simulink model "WindowsiCreateNew"  (R2013a)
settings: Solver=ode3  StartTime=0.0  StopTime=inf  FixedStep=0.01  RelTol=1e-3
undefined symbols (not defined in the file): serial
libraries: instrumentlib x2, vrlib x1, aerolibanimutils x1
settings Model: Creator=Admin  LastModifiedBy=Admin

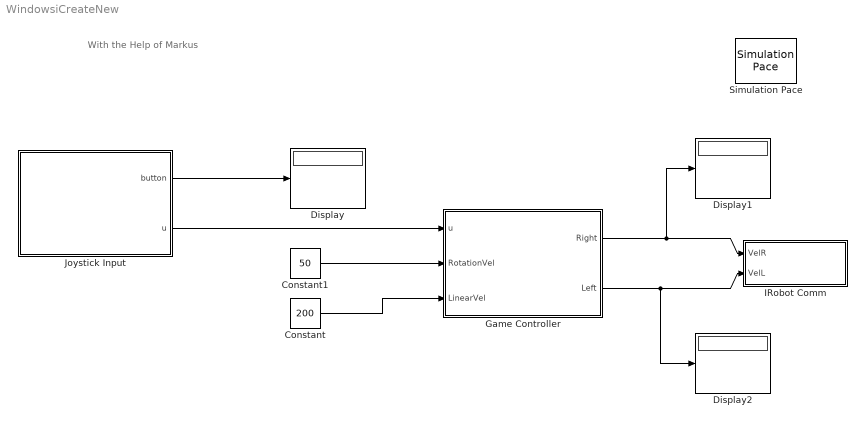
== system WindowsiCreateNew ==
  note: With the Help of Markus
  Constant : Constant  Value=200
  Constant1 : Constant  Value=50
  Display : Display
  Display1 : Display
  Display2 : Display
  Game Controller : MATLAB Function  TreatAsAtomicUnit=on
  IRobot Comm : Subsystem
  Joystick Input : Subsystem
  Simulation Pace : aerolibanimutils/Simulation Pace  SimulationPace=1  SleepMode=MATLAB Thread  OutputPaceError=off  SampleTime=-1
      settings: AttributesFormatString=%<SimulationPace> sec/sec
  wires:
  Joystick Input/1(button) -> Display/1
  Joystick Input/2(u) -> Game Controller/1(u)
  Game Controller/1(Right) -> Display1/1, IRobot Comm/1(VelR)
  Game Controller/2(Left) -> Display2/1, IRobot Comm/2(VelL)
  Constant1/1 -> Game Controller/2(RotationVel)
  Constant/1 -> Game Controller/3(LinearVel)

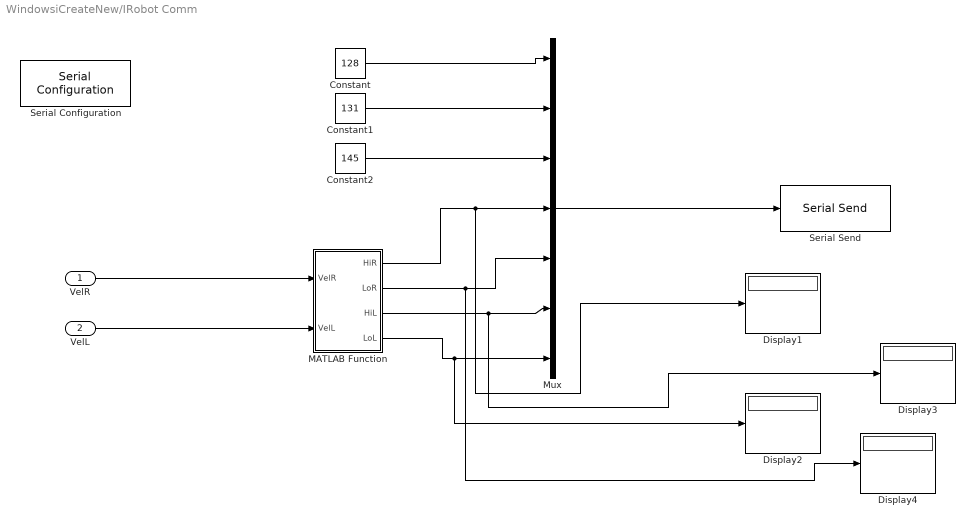
== system WindowsiCreateNew/IRobot Comm ==
  VelR : Inport
  VelL : Inport  Port=2
  Constant : Constant  Value=128  OutDataTypeStr=uint8
  Constant1 : Constant  Value=131  OutDataTypeStr=uint8
  Constant2 : Constant  Value=145  OutDataTypeStr=uint8
  Display{1..4} (4 alike) : Display
  MATLAB Function : MATLAB Function  TreatAsAtomicUnit=on
  Mux : Mux  Inputs=7
  Serial Configuration : instrumentlib/Serial Configuration  Priority=-200000  ComPortMenu=<Please select a port...>  ComPort=COM4  ObjConstructor=serial('COM4');  BaudRate=57600  DataBits=8  Parity=none  StopBits=1  FlowControl=none  Timeout=10  ByteOrder=LittleEndian
  Serial Send : instrumentlib/Serial Send  ComPortMenu=<Please select a port...>  ComPort=COM4  ObjConstructor=serial('COM4');  Terminator=<none>  EnableBlockingMode=off
  wires:
  MATLAB Function/1(HiR) -> Display1/1, Mux/4
  MATLAB Function/2(LoR) -> Display4/1, Mux/5
  MATLAB Function/3(HiL) -> Display3/1, Mux/6
  MATLAB Function/4(LoL) -> Display2/1, Mux/7
  Mux/1 -> Serial Send/1
  VelR/1 -> MATLAB Function/1(VelR)
  VelL/1 -> MATLAB Function/2(VelL)
  Constant/1 -> Mux/1
  Constant1/1 -> Mux/2
  Constant2/1 -> Mux/3

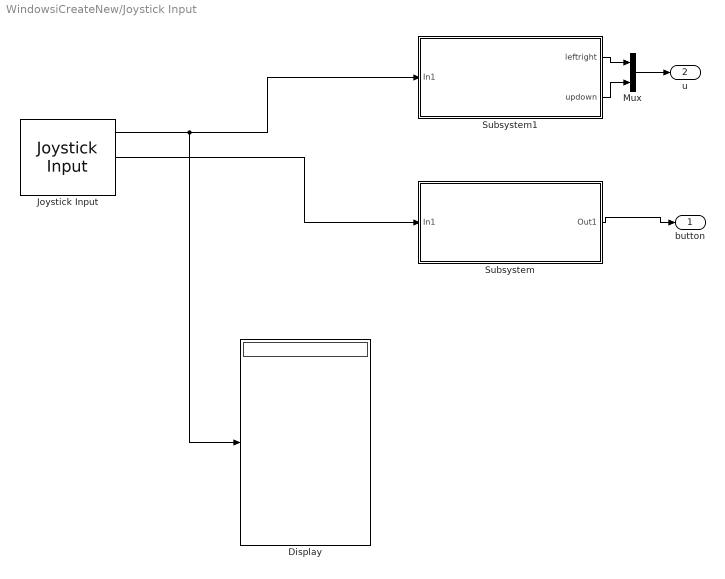
== system WindowsiCreateNew/Joystick Input ==
  Display : Display
  Joystick Input : vrlib/Joystick Input  joyid=1  adjustports=on  forcefeed=off
  Mux : Mux  Inputs=2
  Subsystem : Subsystem
  Subsystem1 : Subsystem
  button : Outport
  u : Outport  Port=2
  wires:
  Subsystem/1(Out1) -> button/1
  Mux/1 -> u/1
  Subsystem1/1(leftright) -> Mux/1
  Subsystem1/2(updown) -> Mux/2
  Joystick Input/1 -> Subsystem1/1(In1), Display/1
  Joystick Input/2 -> Subsystem/1(In1)

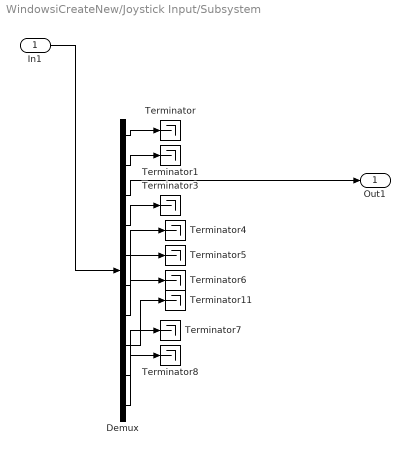
== system WindowsiCreateNew/Joystick Input/Subsystem ==
  In1 : Inport
  Demux : Demux  Outputs=10
  Terminator{,1,3..8,11} (9 alike) : Terminator
  Out1 : Outport
  wires:
  In1/1 -> Demux/1
  Demux/1 -> Terminator/1
  Demux/2 -> Terminator1/1
  Demux/3 -> Out1/1
  Demux/4 -> Terminator3/1
  Demux/5 -> Terminator4/1
  Demux/9 -> Terminator7/1
  Demux/10 -> Terminator8/1
  Demux/6 -> Terminator5/1
  Demux/7 -> Terminator6/1
  Demux/8 -> Terminator11/1

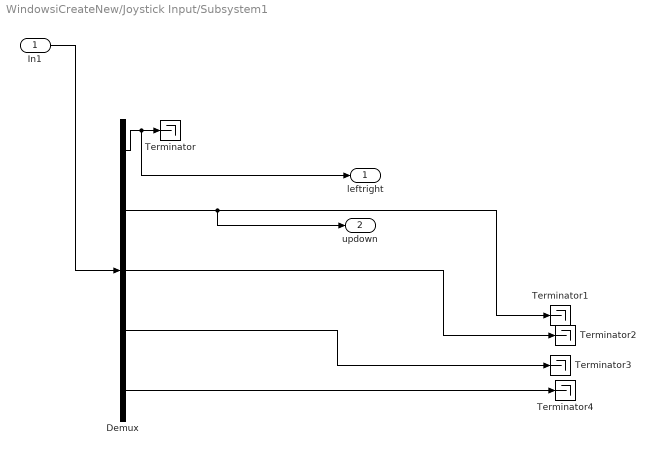
== system WindowsiCreateNew/Joystick Input/Subsystem1 ==
  In1 : Inport
  Demux : Demux  Outputs=5
  Terminator{,1..4} (5 alike) : Terminator
  leftright : Outport
  updown : Outport  Port=2
  wires:
  Demux/5 -> Terminator4/1
  Demux/4 -> Terminator3/1
  Demux/2 -> updown/1, Terminator1/1
  Demux/1 -> leftright/1, Terminator/1
  In1/1 -> Demux/1
  Demux/3 -> Terminator2/1

== matlab function WindowsiCreateNew/Game Controller ==
  data: u input; RotationVel input; LinearVel input; Right output; Left output
function [Right,Left] = fcn(u,RotationVel,LinearVel)
% This block supports the Embedded MATLAB subset.
% See the help menu for details. 

%Converts Joystic commands in velocities
if u(1)==1; %turn right
Right=-RotationVel;
Left=RotationVel;
elseif u(1)==-1;%turn left   
Right=RotationVel;
Left=-RotationVel;
else
Right=0;
Left=0;  
end
    
if u(2)==1; %backwards
Right=-LinearVel+Right;
Left=-LinearVel+Left;
elseif u(2)==-1;%forward   
Right=LinearVel+Right;
Left=LinearVel+Left;
else %stop   
Right=Right;
Left=Left;
end

== matlab function WindowsiCreateNew/IRobot Comm/MATLAB Function ==
  data: VelR input; HiR output; VelL input; LoR output; HiL output; LoL output
function [HiR,LoR,HiL,LoL] = fcn(VelR,VelL)
%#codegen



R=typecast(int16(VelR),'uint8');
 %typecast(int16(-200),'uint8')
 
HiR=R(2);
LoR=R(1);

L=typecast(int16(VelL),'uint8');
 %typecast(int16(-200),'uint8')
 
HiL=L(2);
LoL=L(1);
